simulink model "PID_Controller"  (R2020b)
settings: Solver=VariableStepAuto  StartTime=0.0  StopTime=10  RelTol=1e-3
settings Model: Creator=MY lenovo  LastModifiedBy=MY lenovo
settings DataIOCC: SaveOutput=off  SaveTime=off

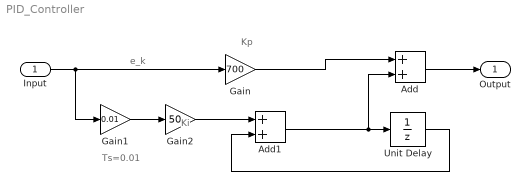
== system PID_Controller ==
  note: Ki
  note: Kp
  note: Ts=0.01
  note: e_k
  Input : Inport  OutDataTypeStr=double  PortDimensions=1  SampleTime=0
  Add : Sum
  Add1 : Sum
  Gain : Gain  Gain=700
  Gain1 : Gain  Gain=0.01
  Gain2 : Gain  Gain=50
  Unit Delay : UnitDelay  SampleTime=-1  HasFrameUpgradeWarning=on
  Output : Outport  OutDataTypeStr=double  PortDimensions=1  SampleTime=0
  wires:
  Input/1 -> Gain/1, Gain1/1
  Gain/1 -> Add/1
  Add/1 -> Output/1
  Gain1/1 -> Gain2/1
  Gain2/1 -> Add1/1
  Add1/1 -> Unit Delay/1, Add/2
  Unit Delay/1 -> Add1/2
